simulink model "Unity_3_Stateflow_Model_Longitudinal"  (R2021a)
settings: Solver=VariableStepAuto  StartTime=0.0  StopTime=100  RelTol=1e-3
libraries: sim3dautolib x2, vrlib x2, simulink x1, mpcadaslib x1, sim3dlib x1
settings Model: Creator=muzaf  LastModifiedBy=muzaf

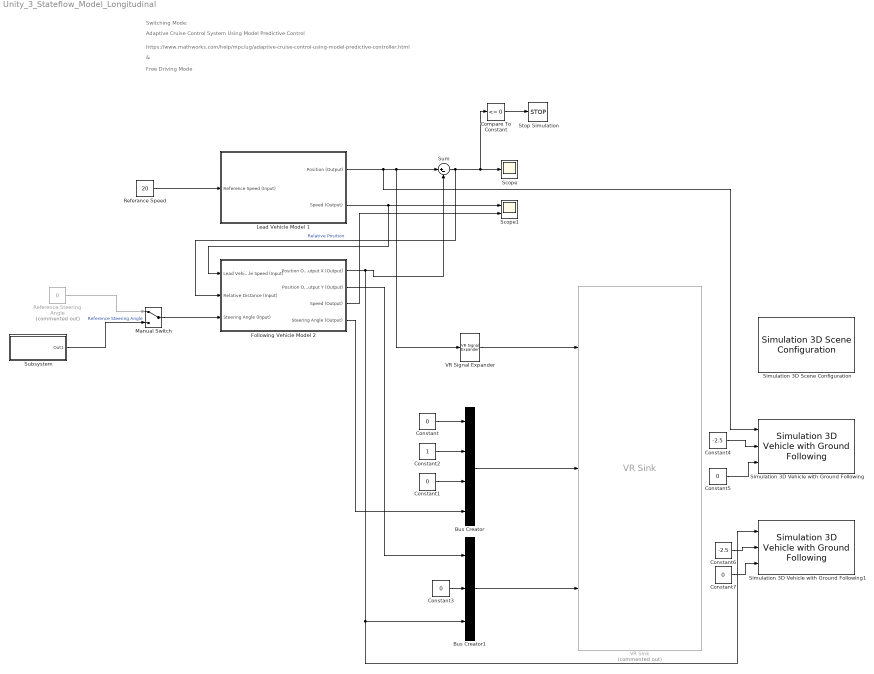
== system Unity_3_Stateflow_Model_Longitudinal ==
  note: Adaptive Cruise Control System Using Model Predictive Control
  note: https://www.mathworks.com/help/mpc/ug/adaptive-cruise-control-using-model-predictive-controller.html
  note: Switching Mode:
  note: &
  note: Free Driving Mode
  Bus Creator : BusCreator  Inputs=4
  Bus Creator1 : BusCreator  Inputs=3
  Compare To Constant : simulink/Logic and Bit Operations/Compare To Constant  relop=<=  const=0  OutDataTypeStr=boolean
  Constant{,1,3,5,7} (5 alike) : Constant  Value=0
  Constant2 : Constant
  Constant4 : Constant  Value=-2.5
  Constant6 : Constant  Value=-2.5
  Following Vehicle Model 2 : Subsystem  mask{Pos=0, Speed=30}
      mask prompts: Pos "Initial Position"; Speed "Initial Speed"
      mask TypeOptions Pos:
      | Initial Position
      | (Constant)/Value
      mask TypeOptions Speed:
      | Initial Speed
      | (Constant)/Value
  Lead Vehicle Model 1 : Subsystem  mask{Pos=35, Speed=15}
      mask prompts: Pos "Initial Position"; Speed "Initial Speed"
      mask TypeOptions Pos:
      | Initial Position
      | (Constant)/Value
      mask TypeOptions Speed:
      | Initial Speed
      | (Constant)/Value
  Manual Switch : ManualSwitch
  Referance Speed : Constant  Value=20
  Reference Steering Angle : Constant  Commented=on  Value=0
  Scope : Scope
  Scope1 : Scope  NumInputPorts=2
  Simulation 3D Scene Configuration : sim3dlib/Simulation 3D Scene Configuration  Priority=0  ProjectFormat=Default Scenes  SceneDesc=Straight road  ProjectName=C:\Program Files\MATLAB\R2021a\toolbox\shared\sim3d_projects\automotive_project\UE4\WindowsNoEditor\VehicleSimulation.exe  ScenePath=/Game/Maps/HwStrght  vehTagList={'Scene Origin';'SimulinkVehicle1';'SimulinkVehicle2'}  vehTag=SimulinkVehicle2  OpVisEn=off  Ts=0.1  EnableWindow=on  EnableWeather=off  SunAltitude=40.0  SunAzimuth=90  clouds=10  wind=1  fog=0  rain=0  sensorTag=MainCamera1  sensorId=1  sensorName=MainCamera1  mountLoc=Origin  offsetFlag=off  tmountOffset=[0, 0, 0]  rmountOffset=[0, 0, 0]  HorizontalResolution=1280  VerticalResolution=720  HorizontalFOV=60  mountPoint=[0 0 0]  mountOrientation=[0 0 0]  aMode=3  ID=1
      settings: SourceProductBaseCode=DR,UV,VE
  Simulation 3D Vehicle with Ground Following : sim3dautolib/Simulation 3D Vehicle with Ground Following  Priority=-1  PassVehMesh=Sedan  MeshPath=/MathWorksSimulation/Vehicles/Muscle/Meshes/SK_MuscleCar.SK_MuscleCar  TrackWidth=1.9  WheelBase=3  WheelRadius=0.35  VehColor=Silver  InitialPos=[0, 0, 0]  InitialRot=[0, 0, 0]  ActorName=SimulinkVehicle1  SampleTime=0.1  ActorType=SimulinkVehicle  ID=1  aMode=3  ActorTag=SimulinkVehicle1  CoordinateScheme=ISO  VehLightsControl=off  HeadlightColor=[ 1, 1, 1 ]  HighBeamIntensity=100000  LowBeamIntensity=60000  HighBeamConeAngle=70  LowBeamConeAngle=70  LeftHeadlightOrientation=[ 0, 0 ]  RightHeadlightOrientation=[ 0, 0 ]  BrakelightIntensity=500  ReverselightIntensity=500  SignallightIntensity=500  SignallightPeriod=1  SignalPulseWidth=50  TransformOutportEnabled=off
      settings: SourceProductBaseCode=DR,UV,VE
  Simulation 3D Vehicle with Ground Following1 : sim3dautolib/Simulation 3D Vehicle with Ground Following  Priority=-1  PassVehMesh=Sedan  MeshPath=/MathWorksSimulation/Vehicles/Muscle/Meshes/SK_MuscleCar.SK_MuscleCar  TrackWidth=1.9  WheelBase=3  WheelRadius=0.35  VehColor=Blue  InitialPos=[0, 0, 0]  InitialRot=[0, 0, 0]  ActorName=SimulinkVehicle2  SampleTime=0.1  ActorType=SimulinkVehicle  ID=2  aMode=3  ActorTag=SimulinkVehicle2  CoordinateScheme=ISO  VehLightsControl=off  HeadlightColor=[ 1, 1, 1 ]  HighBeamIntensity=100000  LowBeamIntensity=60000  HighBeamConeAngle=70  LowBeamConeAngle=70  LeftHeadlightOrientation=[ 0, 0 ]  RightHeadlightOrientation=[ 0, 0 ]  BrakelightIntensity=500  ReverselightIntensity=500  SignallightIntensity=500  SignallightPeriod=1  SignalPulseWidth=50  TransformOutportEnabled=off
      settings: SourceProductBaseCode=DR,UV,VE
  Stop Simulation : Stop
  Subsystem : Subsystem
  Sum : Sum  Inputs=|+-
  VR Signal Expander : vrlib/VR Signal Expander  outwidth=3  outidx=[3]
  VR Sink : vrlib/VR Sink  Commented=on  InstantiateOnLoad=on  SampleTime=0.02  ViewEnable=on  RemoteChange=off  RemoteView=off  FieldsWritten=Car_Red.translation.3.1.1.double#Car_Blue.rotation.4.1.1.double#Car_Blue.translation.3.1.1.double  WorldFileName=PlatoonWorld.WRL  AutoView=off  VideoDimensions=[]  AllowVariableSize=off
  wires:
  Lead Vehicle Model 1/1(Position (Output)) -> Simulation 3D Vehicle with Ground Following/1, VR Signal Expander/1, Sum/1
  Referance Speed/1 -> Lead Vehicle Model 1/1(Reference Speed (Input))
  Following Vehicle Model 2/3(Speed (Output)) -> Scope1/2
  Lead Vehicle Model 1/2(Speed (Output)) -> Following Vehicle Model 2/1(Lead Vehicle Speed (Input)), Scope1/1
  Sum/1 -> Compare To Constant/1, Scope/1, Following Vehicle Model 2/2(Relative Distance (Input))  "Relative Position"
  Compare To Constant/1 -> Stop Simulation/1
  Following Vehicle Model 2/1(Position Output X (Output)) -> Sum/2, Simulation 3D Vehicle with Ground Following1/1, Bus Creator1/3
  VR Signal Expander/1 -> VR Sink/1
  Following Vehicle Model 2/4(Steering Angle (Output)) -> Bus Creator/4
  Constant/1 -> Bus Creator/1
  Constant1/1 -> Bus Creator/3
  Constant2/1 -> Bus Creator/2
  Bus Creator/1 -> VR Sink/2
  Constant3/1 -> Bus Creator1/2
  Bus Creator1/1 -> VR Sink/3
  Following Vehicle Model 2/2(Position Output Y (Output)) -> Bus Creator1/1
  Subsystem/1(Out1) -> Manual Switch/2  "Reference Steering Angle"
  Constant4/1 -> Simulation 3D Vehicle with Ground Following/2
  Constant5/1 -> Simulation 3D Vehicle with Ground Following/3
  Constant6/1 -> Simulation 3D Vehicle with Ground Following1/2
  Constant7/1 -> Simulation 3D Vehicle with Ground Following1/3
  Reference Steering Angle/1 -> Manual Switch/1
  Manual Switch/1 -> Following Vehicle Model 2/3(Steering Angle (Input))

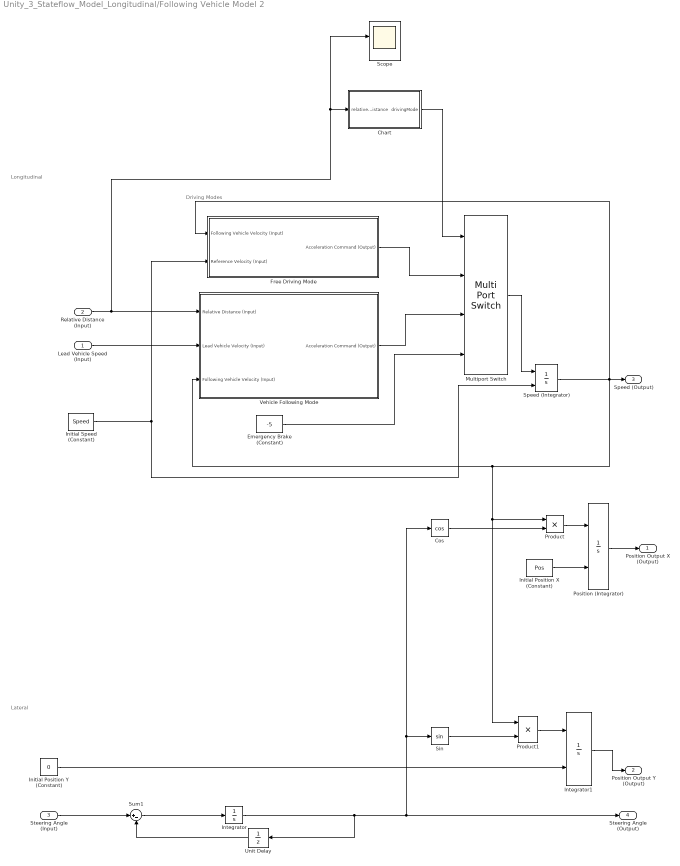
== system Unity_3_Stateflow_Model_Longitudinal/Following Vehicle Model 2 ==
  note: Driving Modes
  note: Lateral
  note: Longitudinal
  Lead Vehicle Speed (Input) : Inport
  Relative Distance (Input) : Inport  Port=2
  Steering Angle (Input) : Inport  Port=3
  Chart : Stateflow chart  TreatAsAtomicUnit=on
  Cos : Trigonometry  Operator=cos
  Emergency Brake (Constant) : Constant  Value=-5
  Free Driving Mode : Subsystem
  Initial Position X (Constant) : Constant  Value=Pos
  Initial Position Y (Constant) : Constant  Value=0
  Initial Speed (Constant) : Constant  Value=Speed
  Integrator : Integrator
  Integrator1 : Integrator  InitialConditionSource=external
  Multiport Switch : MultiPortSwitch
  Position (Integrator) : Integrator  InitialConditionSource=external
  Product : Product
  Product1 : Product
  Scope : Scope  NumInputPorts=4
  Sin : Trigonometry
  Speed (Integrator) : Integrator  InitialConditionSource=external  LimitOutput=on  LowerSaturationLimit=0
  Sum1 : Sum  Inputs=|+-
  Unit Delay : UnitDelay  SampleTime=-1  HasFrameUpgradeWarning=on
  Vehicle Following Mode : Subsystem
  Position Output X (Output) : Outport
  Position Output Y (Output) : Outport  Port=2
  Speed (Output) : Outport  Port=3
  Steering Angle (Output) : Outport  Port=4
  wires:
  Initial Speed (Constant)/1 -> Free Driving Mode/2(Reference Velocity (Input)), Speed (Integrator)/2
  Initial Position X (Constant)/1 -> Position (Integrator)/2
  Speed (Integrator)/1 -> Product1/1, Product/1, Vehicle Following Mode/3(Following Vehicle Velocity (Input)), Speed (Output)/1, Free Driving Mode/1(Following Vehicle Velocity (Input))
  Position (Integrator)/1 -> Position Output X (Output)/1
  Steering Angle (Input)/1 -> Sum1/1
  Sum1/1 -> Integrator/1
  Integrator/1 -> Unit Delay/1, Steering Angle (Output)/1, Sin/1, Cos/1
  Unit Delay/1 -> Sum1/2
  Initial Position Y (Constant)/1 -> Integrator1/2
  Cos/1 -> Product/2
  Product/1 -> Position (Integrator)/1
  Sin/1 -> Product1/2
  Product1/1 -> Integrator1/1
  Integrator1/1 -> Position Output Y (Output)/1
  Relative Distance (Input)/1 -> Scope/2, Chart/1(relativeDistance), Vehicle Following Mode/1(Relative Distance (Input))
  Lead Vehicle Speed (Input)/1 -> Vehicle Following Mode/2(Lead Vehicle Velocity (Input))
  Vehicle Following Mode/1(Acceleration Command (Output)) -> Multiport Switch/3
  Multiport Switch/1 -> Speed (Integrator)/1
  Free Driving Mode/1(Acceleration Command (Output)) -> Multiport Switch/2
  Chart/1(drivingMode) -> Multiport Switch/1
  Emergency Brake (Constant)/1 -> Multiport Switch/4

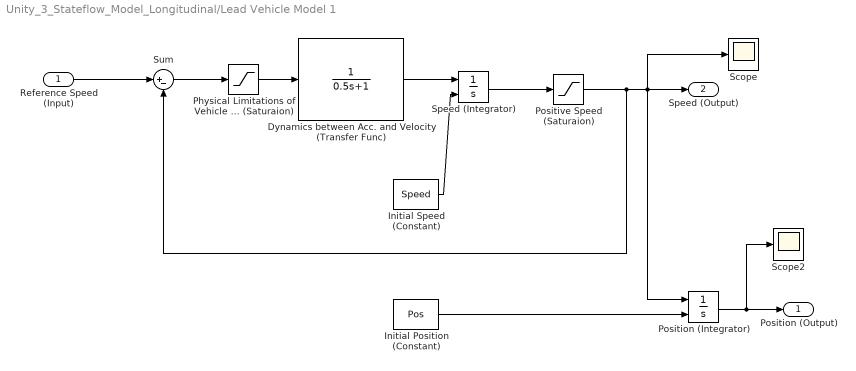
== system Unity_3_Stateflow_Model_Longitudinal/Lead Vehicle Model 1 ==
  Reference Speed (Input) : Inport
  Dynamics between Acc. and Velocity (Transfer Func) : TransferFcn  Denominator=[0.5 1]
  Initial Position (Constant) : Constant  Value=Pos
  Initial Speed (Constant) : Constant  Value=Speed
  Physical Limitations of Vehicle Dynamics Acceleration (Saturaion) : Saturate  UpperLimit=2  LowerLimit=-3
  Position (Integrator) : Integrator  InitialConditionSource=external
  Positive Speed (Saturaion) : Saturate  UpperLimit=inf  LowerLimit=0
  Scope : Scope
  Scope2 : Scope
  Speed (Integrator) : Integrator  InitialConditionSource=external
  Sum : Sum  Inputs=|+-
  Position (Output) : Outport
  Speed (Output) : Outport  Port=2
  wires:
  Physical Limitations of Vehicle Dynamics Acceleration (Saturaion)/1 -> Dynamics between Acc. and Velocity (Transfer Func)/1
  Reference Speed (Input)/1 -> Sum/1
  Position (Integrator)/1 -> Position (Output)/1, Scope2/1
  Dynamics between Acc. and Velocity (Transfer Func)/1 -> Speed (Integrator)/1
  Positive Speed (Saturaion)/1 -> Sum/2, Speed (Output)/1, Position (Integrator)/1, Scope/1
  Initial Position (Constant)/1 -> Position (Integrator)/2
  Sum/1 -> Physical Limitations of Vehicle Dynamics Acceleration (Saturaion)/1
  Speed (Integrator)/1 -> Positive Speed (Saturaion)/1
  Initial Speed (Constant)/1 -> Speed (Integrator)/2

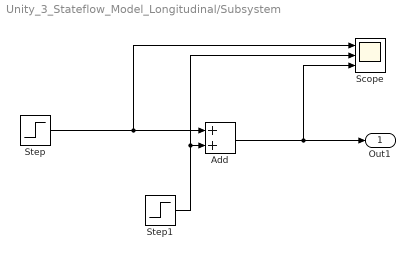
== system Unity_3_Stateflow_Model_Longitudinal/Subsystem ==
  Add : Sum
  Scope : Scope  NumInputPorts=3
  Step : Step  Time=0  After=0.7  SampleTime=0
  Step1 : Step  After=-0.7  SampleTime=0
  Out1 : Outport
  wires:
  Step/1 -> Scope/1, Add/1
  Step1/1 -> Scope/2, Add/2
  Add/1 -> Scope/3, Out1/1

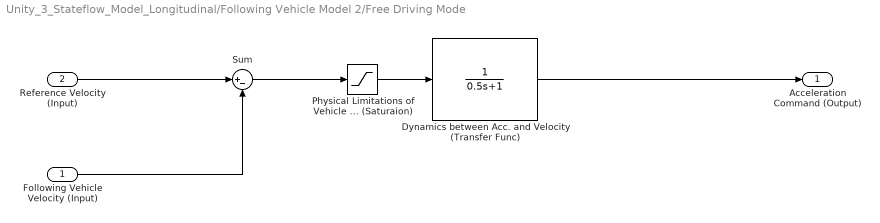
== system Unity_3_Stateflow_Model_Longitudinal/Following Vehicle Model 2/Free Driving Mode ==
  Following Vehicle Velocity (Input) : Inport
  Reference Velocity (Input) : Inport  Port=2
  Dynamics between Acc. and Velocity (Transfer Func) : TransferFcn  Denominator=[0.5 1]
  Physical Limitations of Vehicle Dynamics Acceleration (Saturaion) : Saturate  UpperLimit=2  LowerLimit=-3
  Sum : Sum  Inputs=|+-
  Acceleration Command (Output) : Outport
  wires:
  Reference Velocity (Input)/1 -> Sum/1
  Dynamics between Acc. and Velocity (Transfer Func)/1 -> Acceleration Command (Output)/1
  Sum/1 -> Physical Limitations of Vehicle Dynamics Acceleration (Saturaion)/1
  Physical Limitations of Vehicle Dynamics Acceleration (Saturaion)/1 -> Dynamics between Acc. and Velocity (Transfer Func)/1
  Following Vehicle Velocity (Input)/1 -> Sum/2

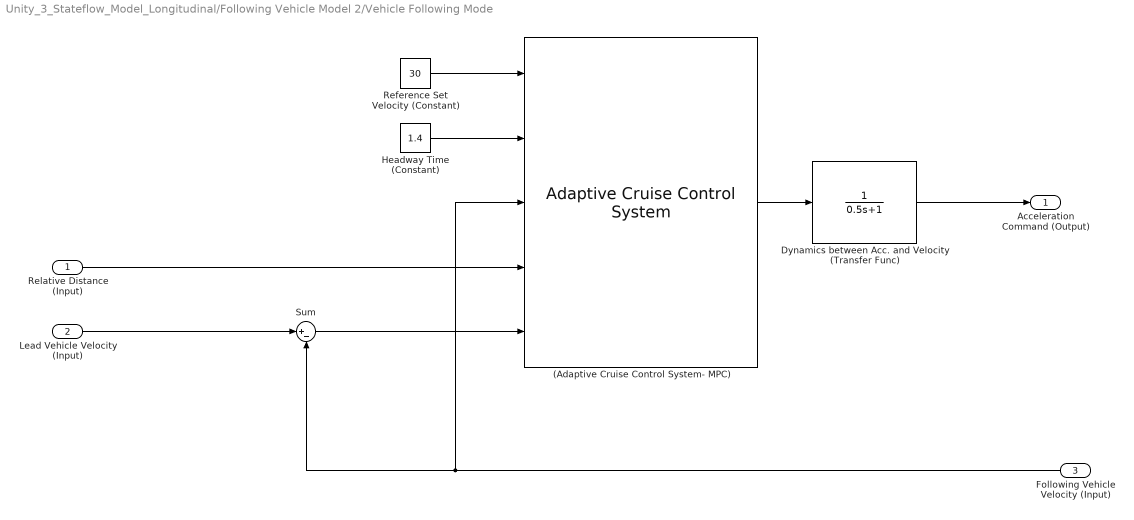
== system Unity_3_Stateflow_Model_Longitudinal/Following Vehicle Model 2/Vehicle Following Mode ==
  Relative Distance (Input) : Inport
  Lead Vehicle Velocity (Input) : Inport  Port=2
  Following Vehicle Velocity (Input) : Inport  Port=3
  (Adaptive Cruise Control System- MPC) : mpcadaslib/Adaptive Cruise Control System  EgoModel=tf(1,[0.5,1,0])  InitialEgoVelocity=30  DefaultSpacing=5  MaxVelocity=50  MinAcceleration=-3  amin_ext=off  MaxAcceleration=2  amax_ext=off  Ts=0.5  PredictionHorizon=200  ControllerBehavior=0.8  suboptimal=off  maxiter=10  datatypeopt=double  optmode=off  trackmode=off
  Dynamics between Acc. and Velocity (Transfer Func) : TransferFcn  Denominator=[0.5 1]
  Headway Time (Constant) : Constant  Value=1.4
  Reference Set Velocity (Constant) : Constant  Value=30
  Sum : Sum  Inputs=|+-
  Acceleration Command (Output) : Outport
  wires:
  Lead Vehicle Velocity (Input)/1 -> Sum/1
  Following Vehicle Velocity (Input)/1 -> Sum/2, (Adaptive Cruise Control System- MPC)/3
  Reference Set Velocity (Constant)/1 -> (Adaptive Cruise Control System- MPC)/1
  (Adaptive Cruise Control System- MPC)/1 -> Dynamics between Acc. and Velocity (Transfer Func)/1
  Headway Time (Constant)/1 -> (Adaptive Cruise Control System- MPC)/2
  Dynamics between Acc. and Velocity (Transfer Func)/1 -> Acceleration Command (Output)/1
  Sum/1 -> (Adaptive Cruise Control System- MPC)/5
  Relative Distance (Input)/1 -> (Adaptive Cruise Control System- MPC)/4

== stateflow chart Unity_3_Stateflow_Model_Longitudinal/Following Vehicle Model 2/Chart ==
  state VehicleFollowing
    entry:
    drivingMode=2;
  state FreeDriving
    entry:
    drivingMode=1;
  state EmergencyBrake
    entry:
    drivingMode=3;
  (default) -> FreeDriving
  FreeDriving -> VehicleFollowing [order 1] : [relativeDistance <= 30]
  VehicleFollowing -> FreeDriving [order 1] : [relativeDistance > 30]
  VehicleFollowing -> EmergencyBrake [order 2] : [relativeDistance <= 10]
  FreeDriving -> EmergencyBrake [order 2] : [relativeDistance <= 10]
  EmergencyBrake -> VehicleFollowing : [relativeDistance > 20]
  data: relativeDistance input; drivingMode output
